simulink library "Pressuredrop"  (R2016b)
settings: Solver=ode45  StartTime=0.0  StopTime=10.0  RelTol=1e-3  EnableMultiTasking=on
settings Model: Creator=lena.frank  LastModifiedBy=drhf
settings DataIOCC: LimitDataPoints=on  SaveFormat=Array  SignalLoggingSaveFormat=ModelDataLogs
settings OptimizationCC: ExpressionDepthLimit=2147483647  LifeSpan=inf
settings DebuggingCC: UnderspecifiedInitializationDetection=Classic  MergeDetectMultiDrivingBlocksExec=none  SolverPrmCheckMsg=warning  FcnCallInpInsideContextMsg=warning  StateNameClashWarn=warning  SFUnexpectedBacktrackingDiag=warning  SFNoUnconditionalDefaultTransitionDiag=warning  SFExecutionAtInitializationDiag=none
settings HardwareCC: ProdBitPerPointer=32  ProdBitPerSizeT=32  ProdBitPerPtrDiffT=32  ProdLargestAtomicFloat=None  ProdIntDivRoundTo=Undefined  ProdEndianess=Unspecified  ProdWordSize=32  ProdHWDeviceType=32-bit Generic
settings ModelReferenceCC: PropagateSignalLabelsOutOfModel=off
settings GRTTargetCC: TargetLangStandard=C89/C90 (ANSI)  GeneratePreprocessorConditionals=Disable all  CombineOutputUpdateFcns=off  GRTInterface=on
settings ConfigComp: CovMetricSettings=dw  CovHtmlReporting=on  CovSaveCumulativeToWorkspaceVar=on  CovSaveSingleToWorkspaceVar=on  CovExternalEMLEnable=off

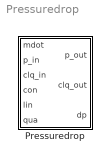
== system Pressuredrop ==
  Pressuredrop : Subsystem  mask(pressure drop){}
      mask help:
      | Pressure drop according to input values of con, lin and qua:
      | dp = con + lin*mdot + qua*mdot²
      | The coefficients are also added to the correponding THB elements.
      mask Help: web(fullfile(path_carnot('help'),'Pressuredrop.html'),'-helpbrowser')

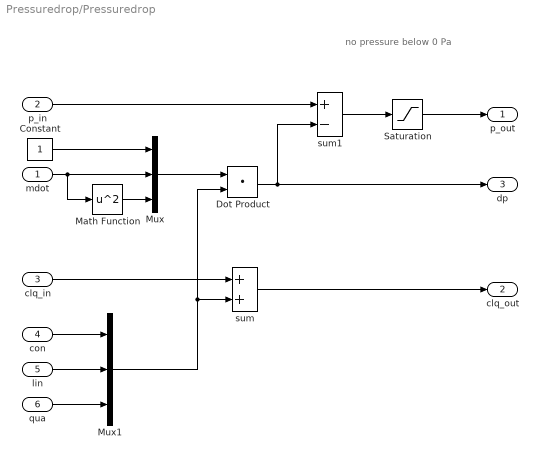
== system Pressuredrop/Pressuredrop ==
  note: no pressure below 0 Pa
  mdot : Inport
  p_in : Inport  Port=2
  clq_in : Inport  Port=3
  con : Inport  Port=4
  lin : Inport  Port=5
  qua : Inport  Port=6
  Constant : Constant
  Dot Product : DotProduct  InputSameDT=on  OutDataTypeStr=Inherit: Inherit via internal rule
  Math Function : Math  Operator=square  SaturateOnIntegerOverflow=on
  Mux : Mux  Inputs=3
  Mux1 : Mux  Inputs=3
  Saturation : Saturate  UpperLimit=inf  LowerLimit=0
  sum : Sum  SaturateOnIntegerOverflow=on  InputSameDT=on  OutDataTypeStr=Inherit: Same as first input
  sum1 : Sum  Inputs=+-  SaturateOnIntegerOverflow=on  InputSameDT=on  OutDataTypeStr=Inherit: Same as first input
  p_out : Outport
  clq_out : Outport  Port=2
  dp : Outport  Port=3
  wires:
  Saturation/1 -> p_out/1
  Constant/1 -> Mux/1
  mdot/1 -> Mux/2, Math Function/1
  Math Function/1 -> Mux/3
  Mux/1 -> Dot Product/1
  con/1 -> Mux1/1
  lin/1 -> Mux1/2
  qua/1 -> Mux1/3
  clq_in/1 -> sum/1
  sum/1 -> clq_out/1
  Mux1/1 -> sum/2, Dot Product/2
  Dot Product/1 -> sum1/2, dp/1
  p_in/1 -> sum1/1
  sum1/1 -> Saturation/1
